simulink model "l16_ex2_PD"  (R2018b)
settings: Solver=ode45  StartTime=0.0  StopTime=6  MaxStep=1e-4  RelTol=1e-3  AbsTol=1e-3  EnableMultiTasking=on
values from neighbouring files (symbols this model uses):
  Kd = 2    [l16.m]    (also in l18.m = 0.031)
  Kp = Kp_list(k)    [l15.m]    (also in l16.m = 8; l18.m = 0.372)
settings Model: Creator=Joe  LastModifiedBy=joema
settings SolverCC: AutoScaleAbsTol=off
settings DataIOCC: LimitDataPoints=on  SaveFormat=Array
settings OptimizationCC: LifeSpan=inf
settings DebuggingCC: UnderspecifiedInitializationDetection=Classic  MergeDetectMultiDrivingBlocksExec=none  LibraryContextMissingDiagnostic=none  SFUnexpectedBacktrackingDiag=warning  SFNoUnconditionalDefaultTransitionDiag=warning  SFExecutionAtInitializationDiag=none
settings HardwareCC: ProdBitPerPointer=32  ProdBitPerSizeT=32  ProdBitPerPtrDiffT=32  ProdLargestAtomicFloat=None  ProdIntDivRoundTo=Undefined  ProdEndianess=Unspecified  ProdWordSize=32  ProdHWDeviceType=32-bit Generic
settings ModelReferenceCC: PropagateSignalLabelsOutOfModel=off
settings SFSimCC: SimUseLocalCustomCode=off
settings RTWCC: RTWUseLocalCustomCode=off
settings CodeAppCC: StateflowObjectComments=on
settings GRTTargetCC: TargetLangStandard=C89/C90 (ANSI)  GeneratePreprocessorConditionals=Disable all
settings ConfigComp: CovMetricSettings=dw  CovHtmlReporting=on  CovSaveCumulativeToWorkspaceVar=on  CovSaveSingleToWorkspaceVar=on  CovExternalEMLEnable=off  CovSFcnEnable=off

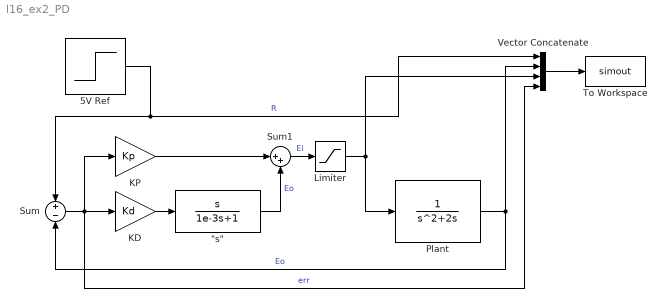
== system l16_ex2_PD ==
  "\"s\"" : TransferFcn  Numerator=[1 0]  Denominator=[1e-3 1]
  5V Ref : Step  Time=0  After=5  SampleTime=0
  KD : Gain  Gain=Kd
  KP : Gain  Gain=Kp
  Limiter : Saturate  UpperLimit=1e4  LowerLimit=-1e4
  Plant : TransferFcn  Numerator=1  Denominator=[1 2 0 ]
  Sum : Sum  Inputs=+-
  Sum1 : Sum  Inputs=|++
  To Workspace : ToWorkspace  VariableName=simout  SaveFormat=Timeseries  SampleTime=-1
  Vector Concatenate : Concatenate  NumInputs=4
  wires:
  5V Ref/1 -> Vector Concatenate/1, Sum/1  "R"
  Sum/1 -> Vector Concatenate/4, KD/1, KP/1  "err"
  Plant/1 -> Sum/2, Vector Concatenate/2  "Eo"
  Vector Concatenate/1 -> To Workspace/1
  KD/1 -> "\"s\""/1
  KP/1 -> Sum1/1
  "\"s\""/1 -> Sum1/2  "Eo"
  Sum1/1 -> Limiter/1  "Ei"
  Limiter/1 -> Plant/1, Vector Concatenate/3
